simulink model "punto5sim"  (R2015a)
settings: Solver=ode45  StartTime=0.0  StopTime=6  RelTol=1e-3
settings Model: Creator=carma_000  LastModifiedBy=carma_000

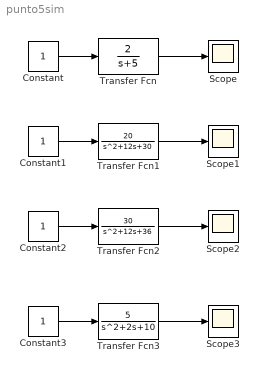
== system punto5sim ==
  Constant{,1..3} (4 alike) : Constant
  Scope{,1..3} (4 alike) : Scope
      Scope2 settings: SaveName=ScopeData2
      Scope3 settings: SaveName=ScopeData3
  Transfer Fcn : TransferFcn  Numerator=[2]  Denominator=[1 5]
  Transfer Fcn1 : TransferFcn  Numerator=[20]  Denominator=[1 12 30]
  Transfer Fcn2 : TransferFcn  Numerator=[30]  Denominator=[1 12 36]
  Transfer Fcn3 : TransferFcn  Numerator=[5]  Denominator=[1 2 10]
  wires:
  Constant/1 -> Transfer Fcn/1
  Transfer Fcn/1 -> Scope/1
  Constant1/1 -> Transfer Fcn1/1
  Transfer Fcn1/1 -> Scope1/1
  Constant2/1 -> Transfer Fcn2/1
  Transfer Fcn2/1 -> Scope2/1
  Constant3/1 -> Transfer Fcn3/1
  Transfer Fcn3/1 -> Scope3/1
